simulink model "mux_test"  (Simulink 7.2)
settings: Solver=ode45  StartTime=0.0  StopTime=10.0  RelTol=1e-3
settings Model: Creator=arnaud  LastModifiedBy=arnaud

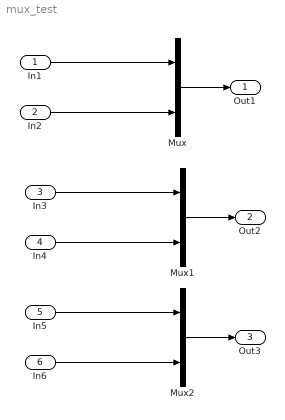
== system mux_test ==
  In1 : Inport  OutDataType=sfix(16)  OutScaling=2^0
  In2 : Inport  Port=2  OutDataType=sfix(16)  OutScaling=2^0
  In3 : Inport  Port=3  OutDataType=sfix(16)  OutScaling=2^0
  In4 : Inport  Port=4  PortDimensions=3  OutDataType=sfix(16)  OutScaling=2^0
  In5 : Inport  Port=5  PortDimensions=2  OutDataType=sfix(16)  OutScaling=2^0
  In6 : Inport  Port=6  PortDimensions=3  OutDataType=sfix(16)  OutScaling=2^0
  Mux : Mux  Inputs=2
  Mux1 : Mux  Inputs=2
  Mux2 : Mux  Inputs=2
  Out1 : Outport  OutDataType=sfix(16)  OutScaling=2^0
  Out2 : Outport  Port=2  OutDataType=sfix(16)  OutScaling=2^0
  Out3 : Outport  Port=3  OutDataType=sfix(16)  OutScaling=2^0
  wires:
  Mux/1 -> Out1/1
  In1/1 -> Mux/1
  In2/1 -> Mux/2
  Mux1/1 -> Out2/1
  In3/1 -> Mux1/1
  In4/1 -> Mux1/2
  Mux2/1 -> Out3/1
  In5/1 -> Mux2/1
  In6/1 -> Mux2/2
